simulink model "NavigationModeA"  (R2025a)
settings: Solver=FixedStepAuto  StartTime=0.0  StopTime=inf  FixedStep=0.01  RelTol=1e-3
model workspace (MAT data in the model file):
  SL_ROS_VariableLengthArrays_MaxSizes.CommonInfo.ArrayTruncateAction = 'EmitWarning'
  SL_ROS_VariableLengthArrays_MaxSizes.MsgTypeMap = containers.Map
  SL_ROS_VariableLengthArrays_MaxSizes.MsgTypeMap.serialization.keys = {'sensor_msgs/Image', 'sensor_msgs/PointCloud2'}
  SL_ROS_VariableLengthArrays_MaxSizes.MsgTypeMap.serialization.values{1}(1).PropertyName = 'Data'
  SL_ROS_VariableLengthArrays_MaxSizes.MsgTypeMap.serialization.values{1}(1).DataType = 'uint8'
  SL_ROS_VariableLengthArrays_MaxSizes.MsgTypeMap.serialization.values{1}(1).MaxLength = 50000000
  SL_ROS_VariableLengthArrays_MaxSizes.MsgTypeMap.serialization.values{1}(2).PropertyName = 'Encoding'
  SL_ROS_VariableLengthArrays_MaxSizes.MsgTypeMap.serialization.values{1}(2).DataType = 'uint8'
  SL_ROS_VariableLengthArrays_MaxSizes.MsgTypeMap.serialization.values{1}(2).MaxLength = 50000000
  SL_ROS_VariableLengthArrays_MaxSizes.MsgTypeMap.serialization.values{2}(1).PropertyName = 'Data'
  SL_ROS_VariableLengthArrays_MaxSizes.MsgTypeMap.serialization.values{2}(1).DataType = 'uint8'
  SL_ROS_VariableLengthArrays_MaxSizes.MsgTypeMap.serialization.values{2}(1).MaxLength = 90000000
  SL_ROS_VariableLengthArrays_MaxSizes.MsgTypeMap.serialization.values{2}(2).PropertyName = 'Fields'
  SL_ROS_VariableLengthArrays_MaxSizes.MsgTypeMap.serialization.values{2}(2).DataType = 'sensor_msgs/PointField'
  SL_ROS_VariableLengthArrays_MaxSizes.MsgTypeMap.serialization.values{2}(2).MaxLength = 16
  SL_ROS_VariableLengthArrays_MaxSizes.MsgTypeMap.serialization.uniformity = 0
  SL_ROS_VariableLengthArrays_MaxSizes.MsgTypeMap.serialization.keyType = 'char'
  SL_ROS_VariableLengthArrays_MaxSizes.MsgTypeMap.serialization.valueType = 'any'
undefined symbols (not defined in the file or in its folder): Drive, gray, X, Y
libraries: robotlib x9
settings Model: Creator=jzx  LastModifiedBy=li
settings SolverCC: AlgebraicLoopSolver=TrustRegion
settings OptimizationCC: EnhancedBackFolding=on  PassReuseOutputArgsAs=Individual arguments  ZeroExternalMemoryAtStartup=off  ZeroInternalMemoryAtStartup=off  MaxStackSize=64  OptimizeBlockOrder=speed  DifferentSizesBufferReuse=on  OptimizationCustomize=off  EfficientTunableParamExpr=on
settings DebuggingCC: ParameterTunabilityLossMsg=error  UnconnectedInputMsg=warning  UnconnectedOutputMsg=warning  UnconnectedLineMsg=warning
settings HardwareCC: ProdBitPerPointer=32.0  ProdBitPerSizeT=32.0  ProdBitPerPtrDiffT=32.0  ProdLargestAtomicFloat=None  ProdIntDivRoundTo=Undefined  ProdEndianess=Unspecified  ProdWordSize=32.0  ProdHWDeviceType=Generic->Unspecified (assume 32-bit Generic)
settings ModelReferenceCC: EnableRefExpFcnMdlSchedulingChecks=on
settings SFSimCC: MATLABDynamicMemAlloc=off
settings RTWCC: SystemTargetFile=ert.tlc  HardwareBoard=Robot Operating System (ROS)  TLCOptions="-aInlineSetEventsForThisBaseRateFcn=TLC_FALSE -aSuppressMultiTaskScheduler=TLC_FALSE  -aRateBasedStepFcn=0"  TemplateMakefile=ert_default_tmf  Toolchain=Catkin  TargetLang=C++  GPUComputeCapability=3.5  DLArmComputeVersion=19.05  Description=Embedded Coder
settings CodeAppCC: ForceParamTrailComments=on  IgnoreCustomStorageClasses=off  OperatorAnnotations=on  SimulinkDataObjDesc=on  SFDataObjDesc=on  InsertBlockDesc=on
settings ERTTargetCC: ExtModeTransport=0.0  ExtModeStaticAlloc=off  ExtModeMexFile=ext_comm  ExtModeIntrfLevel=Level1  InlinedParameterPlacement=Hierarchical  DynamicArrayContainerType=coder::array

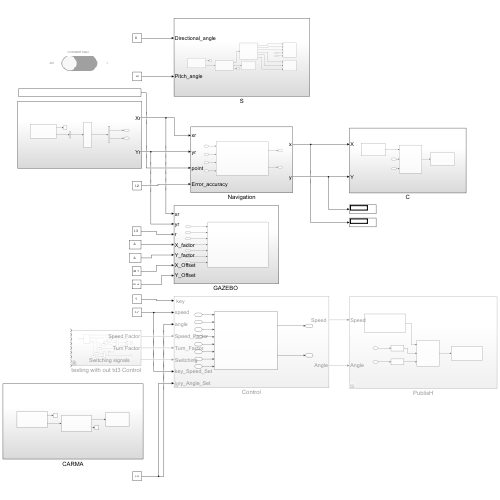
[thumbnail: Simulink's stored preview of the top-level diagram]
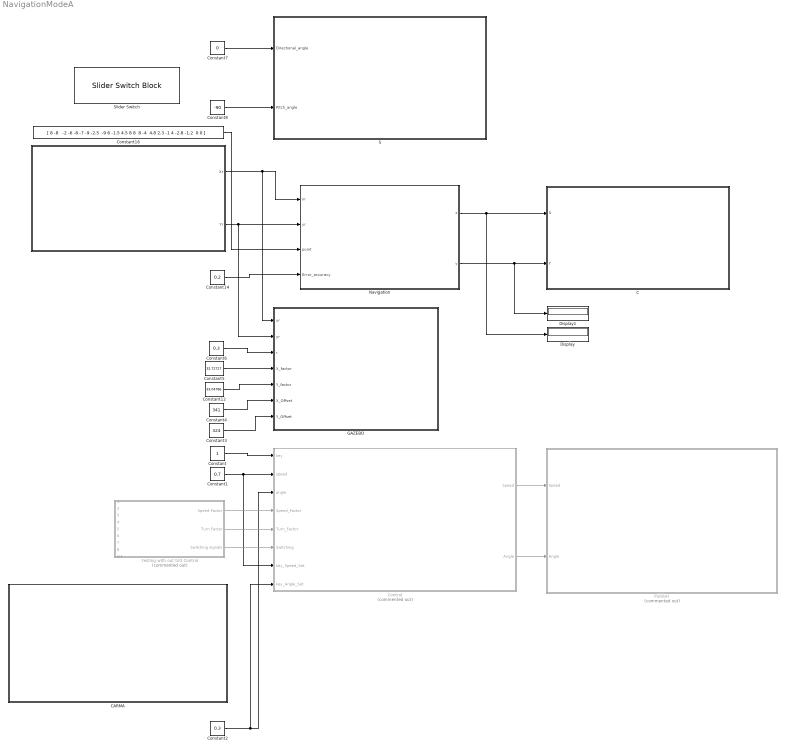
== system NavigationModeA ==
  " " : Subsystem
  C : Subsystem
  CARMA : Subsystem
  Constant : Constant
  Constant1 : Constant  Value=0.7
  Constant12 : Constant  Value=33.04786
  Constant14 : Constant  Value=0.2
  Constant16 : Constant  Value=|
      | [ 8 -8   -2 -6 -8 -7 -9 -2.5  -9 6 -1.5 4.5 8 8  8 -4  4.8 2.3 -1 4 -2.8 -1.2  0 0
      | ]
  Constant2 : Constant  Value=0.3
  Constant3 : Constant  Value=324
  Constant4 : Constant  Value=341
  Constant5 : Constant  Value=32.72727
  Constant6 : Constant  Value=0.3
  Constant7 : Constant  Value=0
  Constant8 : Constant  Value=-90
  Control : Subsystem  Commented=on
  Display : Display
  Display1 : Display
  "GAZEBO " : Subsystem
  Navigation : Subsystem
  PublisH : Subsystem  Commented=on
  S : Subsystem
  Slider Switch : SliderSwitchBlock
  "testing with out td3 Control " : Subsystem  Commented=on
  wires:
  Constant3/1 -> "GAZEBO "/7(Y_Offset)
  Constant7/1 -> S/1(Directional_angle)
  Constant16/1 -> Navigation/3(point)
  Constant5/1 -> "GAZEBO "/4(X_factor)
  Constant2/1 -> Control/8(key_Angle_Set), Control/3(angle)
  Constant4/1 -> "GAZEBO "/6(X_Offset)
  Constant8/1 -> S/2(Pitch_angle)
  Constant6/1 -> "GAZEBO "/3(r)
  " "/2(Yr) -> "GAZEBO "/2(yr), Navigation/2(yr)
  " "/1(Xr) -> "GAZEBO "/1(xr), Navigation/1(xr)
  Constant1/1 -> Control/7(key_Speed_Set), Control/2(speed)
  Constant14/1 -> Navigation/4(Error_accuracy)
  Constant/1 -> Control/1(" key")
  Constant12/1 -> "GAZEBO "/5(Y_factor)
  "testing with out td3 Control "/1(Speed Factor) -> Control/4(Speed_Factor)
  "testing with out td3 Control "/2(Turn Factor) -> Control/5(Turn_Factor)
  "testing with out td3 Control "/3("Switching signals ") -> Control/6(Switching)
  Navigation/1(x) -> Display/1, C/1(X)
  Navigation/2(y) -> Display1/1, C/2(Y)
  Control/1("Speed ") -> PublisH/1(Speed)
  Control/2(Angle) -> PublisH/2(Angle)

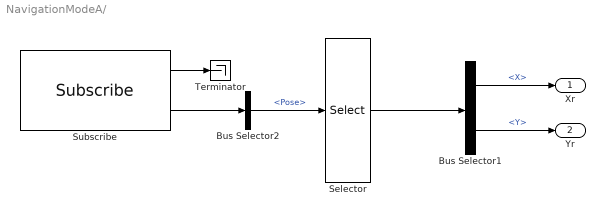
== system NavigationModeA/  ==
  Bus Selector1 : BusSelector  OutputSignals=Position.X,Position.Y
  Bus Selector2 : BusSelector  OutputSignals=Pose
  Selector : Selector  InputPortWidth=16  IndexOptions=Index vector (dialog)  Indices=[2]  OutputSizes=1
  Subscribe : robotlib/Subscribe  topicSource=Select from ROS network  topic=/gazebo/link_states  messageType=gazebo_msgs/LinkStates  SampleTime=-1  legacyBusStruct=off  messageQueueLength=1
  Terminator : Terminator
  Xr : Outport
  Yr : Outport  Port=2
  wires:
  Subscribe/1 -> Terminator/1
  Selector/1 -> Bus Selector1/1
  Subscribe/2 -> Bus Selector2/1
  Bus Selector2/1 -> Selector/1  "<Pose>"
  Bus Selector1/1 -> Xr/1  "<X>"
  Bus Selector1/2 -> Yr/1  "<Y>"

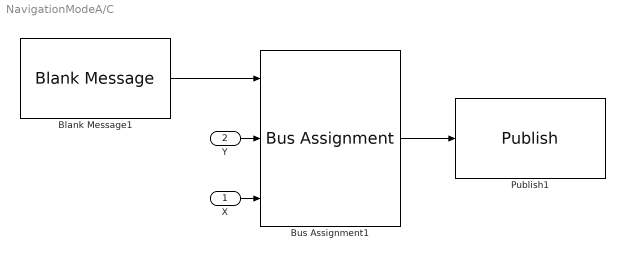
== system NavigationModeA/C ==
  X : Inport
  Y : Inport  Port=2
  Blank Message1 : robotlib/Blank Message  messageClass=Message  entityType=geometry_msgs/Pose2D  messageType=geometry_msgs/Pose2D  SampleTime=inf  legacyBusStruct=off
  Bus Assignment1 : BusAssignment  AssignedSignals=Y,X
  Publish1 : robotlib/Publish  topicSource=Specify your own  topic=/Target_location  messageType=geometry_msgs/Pose2D  legacyBusStruct=off  messageQueueLength=1
  wires:
  Blank Message1/1 -> Bus Assignment1/1
  Bus Assignment1/1 -> Publish1/1
  Y/1 -> Bus Assignment1/2
  X/1 -> Bus Assignment1/3

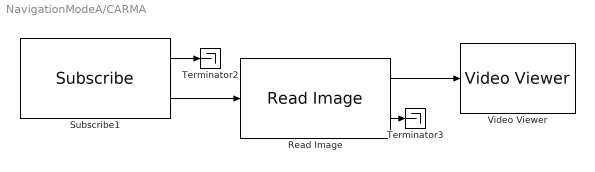
== system NavigationModeA/CARMA ==
  Read Image : robotlib/Read Image  MaximumImageSize=[480, 640]  ImageEncoding=rgb8  ShowAlphaOutput=off  ShowErrorCodeOutput=on  VariableSizeOutputs=off
  Subscribe1 : robotlib/Subscribe  topicSource=Select from ROS network  topic=/camera/image_raw  messageType=sensor_msgs/Image  SampleTime=-1  legacyBusStruct=off  messageQueueLength=1
  Terminator2 : Terminator
  Terminator3 : Terminator
  Video Viewer : VideoViewer  colormapValue=gray(256)  FigPos=[41 738 588 448.8]
  wires:
  Read Image/2 -> Terminator3/1
  Subscribe1/2 -> Read Image/1
  Subscribe1/1 -> Terminator2/1
  Read Image/1 -> Video Viewer/1

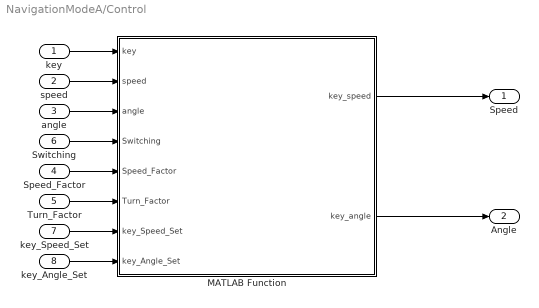
== system NavigationModeA/Control ==
  " key" : Inport
  speed : Inport  Port=2
  angle : Inport  Port=3
  Speed_Factor : Inport  Port=4
  Turn_Factor : Inport  Port=5
  Switching : Inport  Port=6
  key_Speed_Set : Inport  Port=7
  key_Angle_Set : Inport  Port=8
  MATLAB Function : MATLAB Function  TreatAsAtomicUnit=on
  "Speed " : Outport
  Angle : Outport  Port=2
  wires:
  Speed_Factor/1 -> MATLAB Function/5(Speed_Factor)
  Turn_Factor/1 -> MATLAB Function/6(Turn_Factor)
  MATLAB Function/1(key_speed) -> "Speed "/1
  MATLAB Function/2(key_angle) -> Angle/1
  " key"/1 -> MATLAB Function/1(key)
  Switching/1 -> MATLAB Function/4(Switching)
  speed/1 -> MATLAB Function/2(speed)
  angle/1 -> MATLAB Function/3(angle)
  key_Speed_Set/1 -> MATLAB Function/7(key_Speed_Set)
  key_Angle_Set/1 -> MATLAB Function/8(key_Angle_Set)

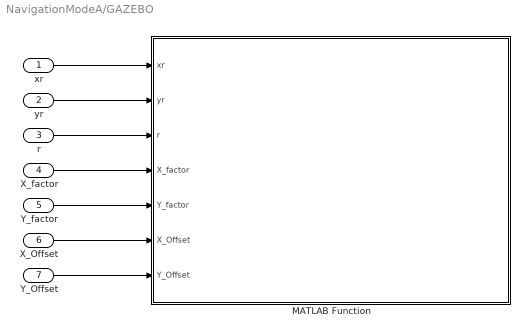
== system NavigationModeA/GAZEBO  ==
  xr : Inport
  yr : Inport  Port=2
  r : Inport  Port=3
  X_factor : Inport  Port=4
  Y_factor : Inport  Port=5
  X_Offset : Inport  Port=6
  Y_Offset : Inport  Port=7
  MATLAB Function : MATLAB Function  TreatAsAtomicUnit=on
  wires:
  Y_Offset/1 -> MATLAB Function/7(Y_Offset)
  X_Offset/1 -> MATLAB Function/6(X_Offset)
  yr/1 -> MATLAB Function/2(yr)
  X_factor/1 -> MATLAB Function/4(X_factor)
  r/1 -> MATLAB Function/3(r)
  Y_factor/1 -> MATLAB Function/5(Y_factor)
  xr/1 -> MATLAB Function/1(xr)

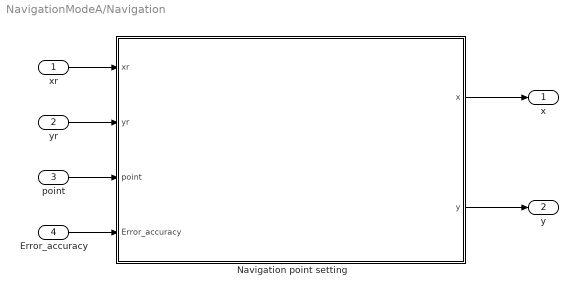
== system NavigationModeA/Navigation ==
  xr : Inport
  yr : Inport  Port=2
  point : Inport  Port=3
  Error_accuracy : Inport  Port=4
  Navigation point setting : MATLAB Function  TreatAsAtomicUnit=on
  x : Outport
  y : Outport  Port=2
  wires:
  Error_accuracy/1 -> Navigation point setting/4(Error_accuracy)
  point/1 -> Navigation point setting/3(point)
  Navigation point setting/2(y) -> y/1
  yr/1 -> Navigation point setting/2(yr)
  xr/1 -> Navigation point setting/1(xr)
  Navigation point setting/1(x) -> x/1

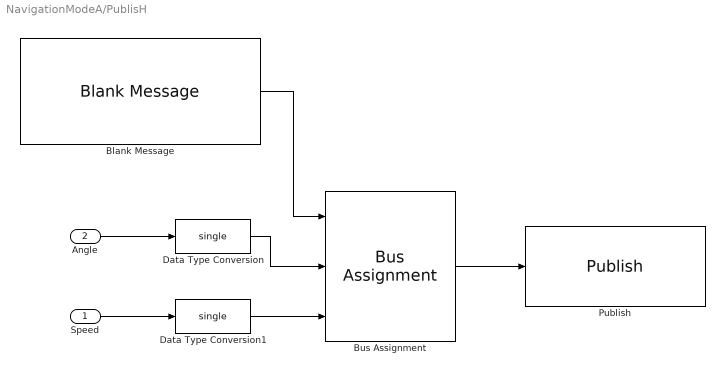
== system NavigationModeA/PublisH ==
  Speed : Inport
  Angle : Inport  Port=2
  Blank Message : robotlib/Blank Message  messageClass=Message  entityType=ackermann_msgs/AckermannDriveStamped  messageType=ackermann_msgs/AckermannDriveStamped  SampleTime=inf  legacyBusStruct=off
  Bus Assignment : BusAssignment  AssignedSignals=Drive.SteeringAngle,Drive.Speed
  Data Type Conversion : DataTypeConversion  OutDataTypeStr=single  SaturateOnIntegerOverflow=off  RndMeth=Floor
  Data Type Conversion1 : DataTypeConversion  OutDataTypeStr=single  SaturateOnIntegerOverflow=off  RndMeth=Floor
  Publish : robotlib/Publish  topicSource=Select from ROS network  topic=/ackermann_cmd_mux/output  messageType=ackermann_msgs/AckermannDriveStamped  legacyBusStruct=off  messageQueueLength=1
  wires:
  Data Type Conversion/1 -> Bus Assignment/2
  Blank Message/1 -> Bus Assignment/1
  Bus Assignment/1 -> Publish/1
  Data Type Conversion1/1 -> Bus Assignment/3
  Angle/1 -> Data Type Conversion/1
  Speed/1 -> Data Type Conversion1/1

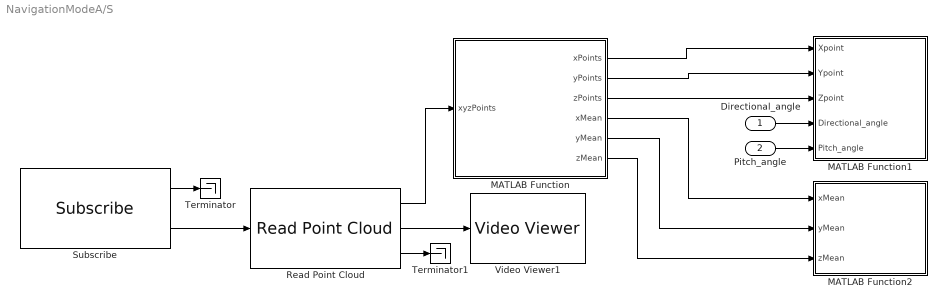
== system NavigationModeA/S ==
  Directional_angle : Inport
  Pitch_angle : Inport  Port=2
  MATLAB Function : MATLAB Function  TreatAsAtomicUnit=on
  MATLAB Function1 : MATLAB Function  TreatAsAtomicUnit=on
  MATLAB Function2 : MATLAB Function  TreatAsAtomicUnit=on
  Read Point Cloud : robotlib/Read Point Cloud  MaximumPointCloudSize=[ 480, 640 ]  PreserveStructure=on  ShowRGBOutput=on  ShowIntensityOutput=off  ShowErrorCodeOutput=on  VariableSizeOutputs=off
  Subscribe : robotlib/Subscribe  topicSource=Select from ROS network  topic=/camera/depth/points  messageType=sensor_msgs/PointCloud2  SampleTime=-1  legacyBusStruct=off  messageQueueLength=1
  Terminator : Terminator
  Terminator1 : Terminator
  Video Viewer1 : VideoViewer  colormapValue=gray(256)  FigPos=[47.4 727.6 576 421.6]
  wires:
  Subscribe/1 -> Terminator/1
  Subscribe/2 -> Read Point Cloud/1
  Read Point Cloud/1 -> MATLAB Function/1(xyzPoints)
  Read Point Cloud/2 -> Video Viewer1/1
  Read Point Cloud/3 -> Terminator1/1
  MATLAB Function/4(xMean) -> MATLAB Function2/1(xMean)
  MATLAB Function/5(yMean) -> MATLAB Function2/2(yMean)
  MATLAB Function/6(zMean) -> MATLAB Function2/3(zMean)
  MATLAB Function/1(xPoints) -> MATLAB Function1/1(Xpoint)
  MATLAB Function/2(yPoints) -> MATLAB Function1/2(Ypoint)
  MATLAB Function/3(zPoints) -> MATLAB Function1/3(Zpoint)
  Directional_angle/1 -> MATLAB Function1/4(Directional_angle)
  Pitch_angle/1 -> MATLAB Function1/5(Pitch_angle)

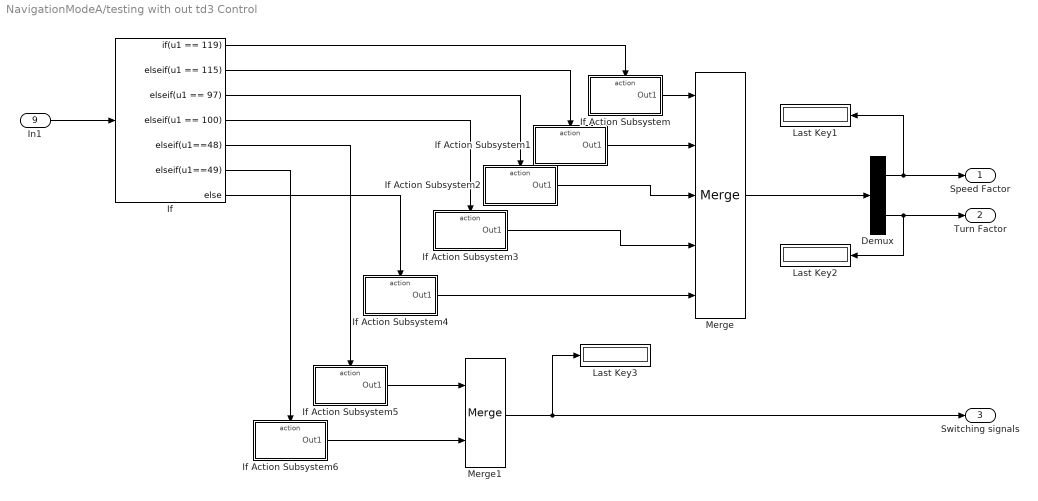
== system NavigationModeA/testing with out td3 Control  ==
  In1 : Inport  Port=9
  Demux : Demux  Outputs=2
  If : If  IfExpression=u1 == 119  ElseIfExpressions=u1 == 115,u1 == 97,u1 == 100 ,u1==48,u1==49
  If Action Subsystem : Subsystem  TreatAsAtomicUnit=on
  If Action Subsystem1 : Subsystem  TreatAsAtomicUnit=on
  If Action Subsystem2 : Subsystem  TreatAsAtomicUnit=on
  If Action Subsystem3 : Subsystem  TreatAsAtomicUnit=on
  If Action Subsystem4 : Subsystem  TreatAsAtomicUnit=on
  If Action Subsystem5 : Subsystem  TreatAsAtomicUnit=on
  If Action Subsystem6 : Subsystem  TreatAsAtomicUnit=on
  Last Key1 : Display
  Last Key2 : Display
  Last Key3 : Display
  Merge : Merge  Inputs=5  InitialOutput=[0 0]
  Merge1 : Merge
  Speed Factor : Outport
  Turn Factor : Outport  Port=2
  "Switching signals " : Outport  Port=3
  wires:
  If/2 -> If Action Subsystem1/Action
  Demux/1 -> Last Key1/1, Speed Factor/1
  If Action Subsystem/1(Out1) -> Merge/1
  If/7 -> If Action Subsystem4/Action
  If Action Subsystem3/1(Out1) -> Merge/4
  If/3 -> If Action Subsystem2/Action
  If Action Subsystem1/1(Out1) -> Merge/2
  If/1 -> If Action Subsystem/Action
  Merge/1 -> Demux/1
  If Action Subsystem4/1(Out1) -> Merge/5
  If/4 -> If Action Subsystem3/Action
  If Action Subsystem2/1(Out1) -> Merge/3
  Demux/2 -> Turn Factor/1, Last Key2/1
  Merge1/1 -> Last Key3/1, "Switching signals "/1
  If Action Subsystem5/1(Out1) -> Merge1/1
  If Action Subsystem6/1(Out1) -> Merge1/2
  If/5 -> If Action Subsystem5/Action
  If/6 -> If Action Subsystem6/Action
  In1/1 -> If/1

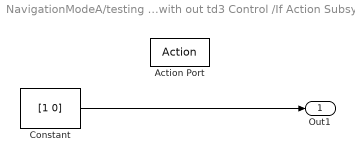
== system NavigationModeA/testing with out td3 Control /If Action Subsystem ==
  Action Port : ActionPort  ActionPortLabel=if(u1 == 119)
  Constant : Constant  Value=[1 0]
  Out1 : Outport
  wires:
  Constant/1 -> Out1/1

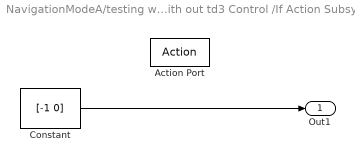
== system NavigationModeA/testing with out td3 Control /If Action Subsystem1 ==
  Action Port : ActionPort  ActionPortLabel=elseif(u1 == 115)
  Constant : Constant  Value=[-1 0]
  Out1 : Outport
  wires:
  Constant/1 -> Out1/1

== system NavigationModeA/testing with out td3 Control /If Action Subsystem2 ==
  Action Port : ActionPort  ActionPortLabel=elseif(u1 == 97)
  Constant : Constant  Value=[1 1]
  Out1 : Outport
  wires:
  Constant/1 -> Out1/1

== system NavigationModeA/testing with out td3 Control /If Action Subsystem3 ==
  Action Port : ActionPort  ActionPortLabel=elseif(u1 == 100 )
  Constant : Constant  Value=[1 -1]
  Out1 : Outport
  wires:
  Constant/1 -> Out1/1

== system NavigationModeA/testing with out td3 Control /If Action Subsystem4 ==
  Action Port : ActionPort  ActionPortLabel=else
  Constant : Constant  Value=[0 0]
  Out1 : Outport
  wires:
  Constant/1 -> Out1/1

== system NavigationModeA/testing with out td3 Control /If Action Subsystem5 ==
  Action Port : ActionPort  ActionPortLabel=elseif(u1==48)
  Constant : Constant
  Out1 : Outport
  wires:
  Constant/1 -> Out1/1

== system NavigationModeA/testing with out td3 Control /If Action Subsystem6 ==
  Action Port : ActionPort  ActionPortLabel=elseif(u1==49)
  Constant : Constant  Value=0
  Out1 : Outport
  wires:
  Constant/1 -> Out1/1

== matlab function NavigationModeA/Navigation/Navigation point setting ==
  data: x output; xr input; y output; yr input; point input; Error_accuracy input
function [x,y] = Navigation_point_setting(xr,yr,point,Error_accuracy)
s=0;
xe=0;
ye=0;
s=size(point,1)/2
persistent i;
if isempty(i)
    i=1;
    
end

x=point(2*i-1);
y=point(2*i);
    
xe=abs(xr-x);
ye=abs(yr-y);
    
if  (xe<=Error_accuracy)&&(ye<=Error_accuracy)
     if  i<s
         i=i+1;
    
     end
end

pause(1)
end

== matlab function NavigationModeA/GAZEBO /MATLAB Function ==
  data: xr input; yr input; r input; X_factor input; Y_factor input; X_Offset input; Y_Offset input
function Gazebo_Track_Plotting(xr,yr,r,X_factor,Y_factor,X_Offset,Y_Offset)
%不要将imshow生成c代码（不支持）
% coder.extrinsic( 'imshow' )
% % 读入图片  
% %Image1=imread('gazebomap.jpg');
% imshow(Image1);
hold on
%计算偏移量
rectangle('Position',[(-yr*X_factor+X_Offset)-r,(-xr*Y_factor+Y_Offset)-r,2*r,2*r],'Curvature',[1,1],'LineWidth',3,'FaceColor','y','EdgeColor','r'),axis equal
end

== matlab function NavigationModeA/Control/MATLAB Function ==
  data: key input; speed input; angle input; Switching input; key_speed output; Speed_Factor input; Turn_Factor input; key_angle output; key_Speed_Set input; key_Angle_Set input
function [key_speed,key_angle] = keys(key,speed,angle,Switching,Speed_Factor,Turn_Factor,key_Speed_Set,key_Angle_Set)
if key==1
   key_speed=Speed_Factor*key_Speed_Set;
   key_angle=Turn_Factor*key_Angle_Set;
else    
   key_speed=(1-Switching)*speed;
   key_angle=(1-Switching)*angle;
end
end

== matlab function NavigationModeA/S/MATLAB Function ==
  data: xPoints output; yPoints output; zPoints output; xyzPoints input; xMean output; yMean output; zMean output
function [xPoints,yPoints,zPoints,xMean,yMean,zMean] = pointCloudCOM(xyzPoints)

% Turn matrix into vectors.
xPoints = reshape(xyzPoints(:,:,1),numel(xyzPoints(:,:,1)),1);
yPoints = reshape(xyzPoints(:,:,2),numel(xyzPoints(:,:,2)),1);
zPoints = reshape(xyzPoints(:,:,3),numel(xyzPoints(:,:,3)),1);

% Calculate the mean for each set of coordinates.
xMean = mean(xPoints,'omitnan');
yMean = mean(yPoints,'omitnan');
zMean = mean(zPoints,'omitnan');

end

== matlab function NavigationModeA/S/MATLAB Function1 ==
  data: Xpoint input; Ypoint input; Zpoint input; Directional_angle input; Pitch_angle input
function fcn(Xpoint,Ypoint,Zpoint,Directional_angle,Pitch_angle)
figure(3)
%不要将imshow生成c代码（不支持）
coder.extrinsic( 'scatter3' )
%plot3(Xpoint,Ypoint,Zpoint)
%plot(Xpoint,Ypoint)
scatter3(Xpoint,Ypoint,Zpoint,'k');
xlabel('x'),ylabel('y'),zlabel('z')
set(gca,'View',[Directional_angle,Pitch_angle]);     %设定视野方向角和俯仰角
end

== matlab function NavigationModeA/S/MATLAB Function2 ==
  data: xMean input; yMean input; zMean input
function fcn(xMean,yMean,zMean)
%不要将imshow生成c代码（不支持）
figure(2)
coder.extrinsic( 'scatter3' )
scatter3(xMean,yMean,zMean,'k');
xlabel('x'),ylabel('y'),zlabel('z')
end
